simulink model "mech_stewart_trajectory"  (R2017a)
settings: Solver=ode45  StartTime=0.0  StopTime=inf  RelTol=1e-3  EnableMultiTasking=on
PreLoadFcn:
  | mech_stewartplatform_dat
PostLoadFcn:
  | find_system(gcs,'FollowLinks', 'on', 'LookUnderMasks', 'all');
InitFcn:
  | find_system(gcs,'FollowLinks', 'on', 'LookUnderMasks', 'all');
undefined symbols (not defined in the file): body_pts, height, Kd, Ki, Kp, lower_leg_mass, pos_base, pos_top, top_inertia, top_mass, upper_leg_mass
libraries: mblibv1 x9, mech_stewartplatform_leg x6
Description:
  | Stewart Platform with Control Reference Trajectory
  | 
  | This example shows a Stewart platform with predefined reference trajectory. A Stewart platform is a six-degree-of-freedom machine for precise positioning and orienting. It consists of a top plate connected to a fixed base through six parallel legs. By extending or shortening the legs and swiveling them on a set of universal joints, the plate's original six degrees of freedom are reproduced with greater stability and precision.
  | 
  | The model is separated into a plant subsystem, the Stewart platform along with necessary actuators and sensors, and a controller subsystem that guides the platform through a predefined motion profile with actuation signals. The controller keeps the actual motion close to the reference motion via sensor-actuator feedback.
  | 
  | 
  | Copyright 2008-2017 The MathWorks, Inc.
settings Model: FPTRunName=Active  ExtModeAutoUpdateStatusClock=off  Creator=MathWorks  LastModifiedBy=smiller
settings DataIOCC: LimitDataPoints=on  SaveFormat=Array  SignalLoggingSaveFormat=ModelDataLogs  SignalLoggingName=logsOut  OutputTimes=[0:0.01:50]
settings OptimizationCC: BooleanDataType=off  ExpressionDepthLimit=2147483647  InitFltsAndDblsToZero=on  LifeSpan=inf
settings DebuggingCC: UnderspecifiedInitializationDetection=Classic  MergeDetectMultiDrivingBlocksExec=none  CheckExecutionContextPreStartOutputMsg=on  CheckExecutionContextRuntimeOutputMsg=on  SignalResolutionControl=TryResolveAllWithWarning  MultiTaskDSMMsg=warning  MultiTaskCondExecSysMsg=none  SigSpecEnsureSampleTimeMsg=none  FcnCallInpInsideContextMsg=warning  StateNameClashWarn=warning  StrictBusMsg=None  SFUnexpectedBacktrackingDiag=warning  SFNoUnconditionalDefaultTransitionDiag=warning  SFExecutionAtInitializationDiag=none
settings HardwareCC: ProdBitPerPointer=32  ProdBitPerSizeT=32  ProdBitPerPtrDiffT=32  ProdLargestAtomicFloat=None  ProdIntDivRoundTo=Undefined  ProdEndianess=Unspecified  ProdWordSize=32  ProdHWDeviceType=32-bit Generic  TargetBitPerPointer=64  TargetBitPerSizeT=64  TargetBitPerPtrDiffT=64  TargetLongLongMode=on  TargetIntDivRoundTo=Zero  TargetEndianess=LittleEndian  TargetWordSize=64  TargetHWDeviceType=MATLAB Host  ProdEqTarget=off
settings ModelReferenceCC: PropagateSignalLabelsOutOfModel=off
settings GRTTargetCC: TargetLangStandard=C89/C90 (ANSI)  GeneratePreprocessorConditionals=Disable all  CombineOutputUpdateFcns=off  GRTInterface=on
settings ConfigComp: CovMetricSettings=dw  CovHtmlReporting=on  CovSaveCumulativeToWorkspaceVar=on  CovSaveSingleToWorkspaceVar=on  CovExternalEMLEnable=off
settings ConfigurationSet: Description=SimMechanics 2G

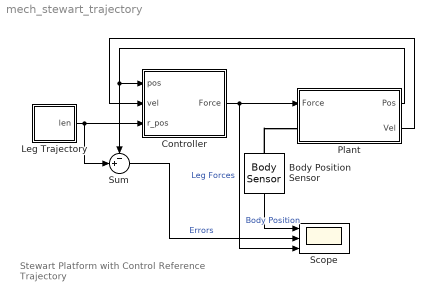
== system mech_stewart_trajectory ==
  note: Stewart Platform
      | with Control Reference Trajectory
  Body Position Sensor : mblibv1/Sensors &  Actuators/Body Sensor  UpdateFromCAD=off  PhysicalDomain=Mechanical  PortType=blob  Muxed=on  Pose=off  Angle=on  AngleUnits=deg  ArcVelocity=off  ArcVelocityUnits=deg/s  ArcAcceleration=off  ArcAccelerationUnits=deg/s^2  CoordPosition=on  CoordPositionUnits=m  Velocity=off  VelocityUnits=m/s  Acceleration=off  AccelerationUnits=m/s^2  Quaternion=on  QuaternionDT=off  QuaternionDDT=off  QuaternionUnits=off  OutputVector=[ 3 ]  ActiveIO=on  Width=3  DialogClass=MechanicalSensorBlock  ReferenceFrame=Absolute (World)
      settings: SourceProductName=Simscape Multibody  SourceProductBaseCode=MS
  Controller : Subsystem
  Leg Trajectory : Subsystem
  Plant : Subsystem
  Scope : Scope  NumInputPorts=3
      settings: Tag=OpenMeAtStartUp
  Sum : Sum  Inputs=-+|  SaturateOnIntegerOverflow=on  InputSameDT=on  OutDataTypeStr=Inherit: Same as first input
  wires:
  Plant/1(Pos) -> Sum/1, Controller/1(pos)
  Controller/1(Force) -> Plant/1(Force), Scope/3  "Leg Forces"
  Body Position Sensor/1 -> Scope/1  "Body Position"
  Sum/1 -> Scope/2  "Errors"
  Leg Trajectory/1(len) -> Controller/3(r_pos), Sum/2
  Plant/2(Vel) -> Controller/2(vel)
  connections:
  Body Position Sensor/LConn1 -- Plant/LConn1

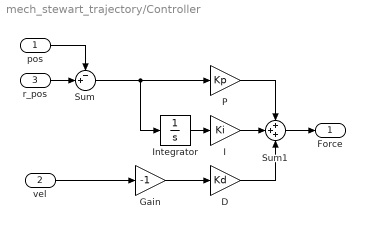
== system mech_stewart_trajectory/Controller ==
  pos : Inport
  vel : Inport  Port=2
  r_pos : Inport  Port=3
  D : Gain  Gain=Kd  SaturateOnIntegerOverflow=on  OutDataTypeStr=Inherit: Same as input  ParamDataTypeStr=Inherit: Same as input
  Gain : Gain  Gain=-1  SaturateOnIntegerOverflow=on  OutDataTypeStr=Inherit: Same as input  ParamDataTypeStr=Inherit: Same as input
  I : Gain  Gain=Ki  SaturateOnIntegerOverflow=on  OutDataTypeStr=Inherit: Same as input  ParamDataTypeStr=Inherit: Same as input
  Integrator : Integrator  InitialCondition=(upper_leg_mass+lower_leg_mass+(top_mass*1.3/6))*9.81/Ki  ZeroCross=off
  P : Gain  Gain=Kp  SaturateOnIntegerOverflow=on  OutDataTypeStr=Inherit: Same as input  ParamDataTypeStr=Inherit: Same as input
  Sum : Sum  Inputs=-+|  SaturateOnIntegerOverflow=on  InputSameDT=on  OutDataTypeStr=Inherit: Same as first input
  Sum1 : Sum  Inputs=+++  SaturateOnIntegerOverflow=on  InputSameDT=on  OutDataTypeStr=Inherit: Same as first input
  Force : Outport
  wires:
  Sum/1 -> P/1, Integrator/1
  I/1 -> Sum1/2
  P/1 -> Sum1/1
  Integrator/1 -> I/1
  vel/1 -> Gain/1
  D/1 -> Sum1/3
  pos/1 -> Sum/1
  Sum1/1 -> Force/1
  r_pos/1 -> Sum/2
  Gain/1 -> D/1

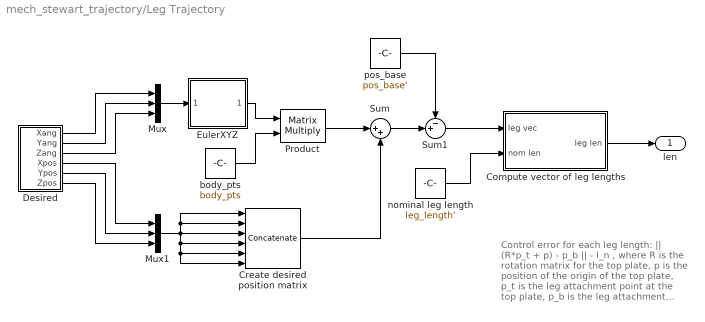
== system mech_stewart_trajectory/Leg Trajectory ==
  note: Control error for each leg length:
      |
      |   || (R*p_t + p) - p_b || - l_n ,
      |
      | where R is the rotation matrix
      | for the top plate, p is the position
      | of the origin of the top plate, p_t
      | is the leg attachment point at the
      | top plate, p_b is the leg attachment
      | point at the base, and l_n is the
      | nominal (reference) distance between
      | the top and base attachment points.
  Compute vector of leg lengths : Subsystem  TreatAsAtomicUnit=on
  Create desired position matrix : Concatenate  NumInputs=6  Mode=Multidimensional array  ConcatenateDimension=2
  Desired : Subsystem
  EulerXYZ : Subsystem  mask(EulerXYZ){}
      mask help: Creates the EulerXYZ rotation matrix corresponding to body fixed rotations in the X, Y, and then Z. This matrix maps body vectors to world vectors.
      mask Help:
      | <p>This block determines the EulerXYZ matrix from a 3x1 euler angles in the X, Y, & Z directions. The matrix maps vectors the body axes to the inertial axes.</p>
      | 
      | <p>The block input and output contain more than one signal as described below.</p>
      | 
      | <p><H4>Block Vector Input - Euler XYZ angles</H4>
      |     <ul>
      |     <li>X angle</li>
      |     <li>Y angle</li>
      |     <li>Z angle</li>
      |    </ul>
      |    </p>
      | 
      | <p><H4>Block Matrix Output - XYZ Euler Matrix </H4>
      |     <ul>
      |    </ul>
      |    </p>
      mask Display: disp('Rotation\nMatrix')
  Mux : Mux  Inputs=3
  Mux1 : Mux  Inputs=3
  Product : Product  Multiplication=Matrix(*)  SaturateOnIntegerOverflow=on  InputSameDT=on  OutDataTypeStr=Inherit: Same as first input
  Sum : Sum  Inputs=|++  SaturateOnIntegerOverflow=on  InputSameDT=on  OutDataTypeStr=Inherit: Same as first input
  Sum1 : Sum  Inputs=-+|  SaturateOnIntegerOverflow=on  InputSameDT=on  OutDataTypeStr=Inherit: Same as first input
  body_pts : Constant  Value=body_pts  VectorParams1D=off
  nominal leg length : Constant  Value=leg_length'  VectorParams1D=off
  pos_base : Constant  Value=pos_base'  VectorParams1D=off
  len : Outport
  wires:
  Mux/1 -> EulerXYZ/1(x y z angles)
  EulerXYZ/1(EulerXYZ) -> Product/1
  body_pts/1 -> Product/2
  Product/1 -> Sum/1
  Mux1/1 -> Create desired position matrix/3, Create desired position matrix/1, Create desired position matrix/2, Create desired position matrix/4, Create desired position matrix/5, Create desired position matrix/6
  Create desired position matrix/1 -> Sum/2
  pos_base/1 -> Sum1/1
  Sum/1 -> Sum1/2
  Sum1/1 -> Compute vector of leg lengths/1(leg vec)
  nominal leg length/1 -> Compute vector of leg lengths/2(nom len)
  Compute vector of leg lengths/1(leg len) -> len/1
  Desired/3(Zang) -> Mux/3
  Desired/1(Xang) -> Mux/1
  Desired/2(Yang) -> Mux/2
  Desired/4(Xpos) -> Mux1/1
  Desired/5(Ypos) -> Mux1/2
  Desired/6(Zpos) -> Mux1/3

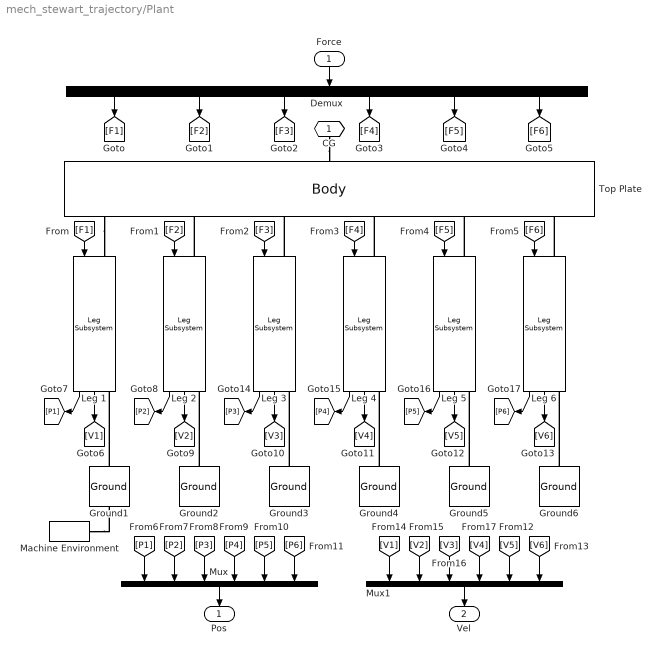
== system mech_stewart_trajectory/Plant ==
  Force : Inport
  Demux : Demux  Outputs=6
  Ground1 : mblibv1/Bodies/Ground  UpdateFromCAD=off  LeftPortType=env  RightPortType=workingframe  PhysicalDomain=Mechanical  DialogClass=GroundBlock  CoordPosition=pos_base(1,:)  CoordPositionUnits=m  StateVectorMgrId=-1  MachineId=[0 0]  ShowEnvPort=on  ParameterChecksum=[0 0 0 0]  TopologyChecksum=[0 0 0 0]
      settings: SourceProductName=Simscape Multibody  SourceProductBaseCode=MS
  Ground2 : mblibv1/Bodies/Ground  UpdateFromCAD=off  LeftPortType=env  RightPortType=workingframe  PhysicalDomain=Mechanical  DialogClass=GroundBlock  CoordPosition=pos_base(2,:)  CoordPositionUnits=m  StateVectorMgrId=-1  MachineId=[0 0]  ShowEnvPort=off  ParameterChecksum=[0 0 0 0]  TopologyChecksum=[0 0 0 0]
      settings: SourceProductName=Simscape Multibody  SourceProductBaseCode=MS
  Ground3 : mblibv1/Bodies/Ground  UpdateFromCAD=off  LeftPortType=env  RightPortType=workingframe  PhysicalDomain=Mechanical  DialogClass=GroundBlock  CoordPosition=pos_base(3,:)  CoordPositionUnits=m  StateVectorMgrId=-1  MachineId=[0 0]  ShowEnvPort=off  ParameterChecksum=[0 0 0 0]  TopologyChecksum=[0 0 0 0]
      settings: SourceProductName=Simscape Multibody  SourceProductBaseCode=MS
  Ground4 : mblibv1/Bodies/Ground  UpdateFromCAD=off  LeftPortType=env  RightPortType=workingframe  PhysicalDomain=Mechanical  DialogClass=GroundBlock  CoordPosition=pos_base(4,:)  CoordPositionUnits=m  StateVectorMgrId=-1  MachineId=[0 0]  ShowEnvPort=off  ParameterChecksum=[0 0 0 0]  TopologyChecksum=[0 0 0 0]
      settings: SourceProductName=Simscape Multibody  SourceProductBaseCode=MS
  Ground5 : mblibv1/Bodies/Ground  UpdateFromCAD=off  LeftPortType=env  RightPortType=workingframe  PhysicalDomain=Mechanical  DialogClass=GroundBlock  CoordPosition=pos_base(5,:)  CoordPositionUnits=m  StateVectorMgrId=-1  MachineId=[0 0]  ShowEnvPort=off  ParameterChecksum=[0 0 0 0]  TopologyChecksum=[0 0 0 0]
      settings: SourceProductName=Simscape Multibody  SourceProductBaseCode=MS
  Ground6 : mblibv1/Bodies/Ground  UpdateFromCAD=off  LeftPortType=env  RightPortType=workingframe  PhysicalDomain=Mechanical  DialogClass=GroundBlock  CoordPosition=pos_base(6,:)  CoordPositionUnits=m  StateVectorMgrId=-1  MachineId=[0 0]  ShowEnvPort=off  ParameterChecksum=[0 0 0 0]  TopologyChecksum=[0 0 0 0]
      settings: SourceProductName=Simscape Multibody  SourceProductBaseCode=MS
  Leg 1 : mech_stewartplatform_leg/Leg Subsystem  ln=1
  Leg 2 : mech_stewartplatform_leg/Leg Subsystem  ln=2
  Leg 3 : mech_stewartplatform_leg/Leg Subsystem  ln=3
  Leg 4 : mech_stewartplatform_leg/Leg Subsystem  ln=4
  Leg 5 : mech_stewartplatform_leg/Leg Subsystem  ln=5
  Leg 6 : mech_stewartplatform_leg/Leg Subsystem  ln=6
  Machine Environment : mblibv1/Bodies/Machine Environment  Tag=Factory ground  PortType=env  PhysicalDomain=Mechanical  DialogTemplateClass=MECH.MachineEnvironment  SyncWhenCopied=off  Gravity=[0 0 -9.81]  GravityUnits=m/s^2  GravityAsSignal=off  Dimensionality=3D Only  AnalysisType=Forward dynamics  LinearAssemblyTolerance=1e-3  LinearAssemblyToleranceUnits=m  AngularAssemblyTolerance=1e-3  AngularAssemblyToleranceUnits=rad  ConstraintSolverType=Machine precision  ConstraintRelTolerance=1e-4  ConstraintAbsTolerance=1e-4  UseRobustSingularityHandling=on  RedundancyAnalysisToleranceType=Automatically select tolerance  RedundancyAnalysisTolerance=1e-14  StatePerturbationType=Adaptive  PerturbationSize=1e-3  VisualizeMachine=on  BodyVisualizationType=Use model default body geometries  BodyColorSelMode=Use model default  DefaultBodyColor=[1 0 0]
      settings: SourceProductName=Simscape Multibody  SourceProductBaseCode=MS
  Mux : Mux  Inputs=6
  Mux1 : Mux  Inputs=6
  Top Plate : mblibv1/Bodies/Body  LConnTagsString=CG  RConnTagsString=CS1|CS2|CS3|CS4|CS5|CS6  UpdateFromCAD=off  DialogClass=MechanicalBodyBlock  Mass=top_mass  MassUnits=kg  InertiaUnits=kg*m^2  Inertia=top_inertia  Shape=Cylinder  ShapeDims=[1 1]  ShapeUnits=m  ShapeUse=false  Density=1  DensityUnits=kg/m^3  DensityUse=false  GraphicsMode=MACHINE_DEFAULT  BodyColorSelMode=MACHINE_DEFAULT  BodyColor=[1 0 0]  AttachedToCS=CG  CG=Left$CG$[0 0 height]$WORLD$WORLD$m$[0 0 0]$Euler X-Y-Z$deg$WORLD$true  WorkingFrames=Right$CS1$pos_top(1,:)$WORLD$WORLD$m$[0 0 0]$Euler X-Y-Z$deg$WORLD$true#Right$CS2$pos_top(2,:)$WORLD$WORLD$m$[0 0 0]$Euler X-Y-Z$deg$WORLD$true#Right$CS3$pos_top(3,:)$WORLD$WORLD$m$[0 0 0]$Euler X-Y-Z$deg$WORLD$true#Right$CS4$pos_top(4,:)$WORLD$WORLD$m$[0 0 0]$Euler X-Y-Z$deg$WORLD$true#Right$CS5$pos_top(5,:)$WORLD$WORLD$m$[0 0 0]$Euler X-Y-Z$deg$WORLD$true#Right$CS6$pos_top(6,:)$WORLD$WORLD$m$[0 0 0]$Euler X-Y-Z$deg$WORLD$true  CGPos=[0 0 height]  CGRot=[0 0 0]  CS0Pos=[]  CS0Rot=[]  CS1Pos=pos_top(1,:)  CS1Rot=[0 0 0]  CS2Pos=pos_top(2,:)  CS2Rot=[0 0 0]  CS3Pos=pos_top(3,:)  CS3Rot=[0 0 0]  CS4Pos=pos_top(4,:)  CS4Rot=[0 0 0]  CS5Pos=pos_top(5,:)  CS5Rot=[0 0 0]  CS6Pos=pos_top(6,:)  CS6Rot=[0 0 0]  CS7Pos=[]  CS7Rot=[]  CS8Pos=[]  CS8Rot=[]  CS9Pos=[]  CS9Rot=[]  CS10Pos=[]  CS10Rot=[]  CS11Pos=[]  CS11Rot=[]  CS12Pos=[]  CS12Rot=[]  CS13Pos=[]  CS13Rot=[]  CS14Pos=[]  CS14Rot=[]  CS15Pos=[]  CS15Rot=[]  CS16Pos=[]  CS16Rot=[]  CS17Pos=[]  CS17Rot=[]  CS18Pos=[]  CS18Rot=[]  CS19Pos=[]  CS19Rot=[]  CS20Pos=[]  CS20Rot=[]
      settings: SourceProductName=Simscape Multibody  SourceProductBaseCode=MS
  CG : PMIOPort  Port=1  Side=Left
  Pos : Outport
  Vel : Outport  Port=2
  wires:
  Force/1 -> Demux/1
  Mux/1 -> Pos/1
  Demux/1 -> [F1]
  Demux/2 -> [F2]
  Demux/3 -> [F3]
  Demux/4 -> [F4]
  Demux/5 -> [F5]
  Demux/6 -> [F6]
  [F1] -> Leg 1/1
  [F2] -> Leg 2/1
  [F3] -> Leg 3/1
  [F4] -> Leg 4/1
  [F5] -> Leg 5/1
  [F6] -> Leg 6/1
  Leg 1/2 -> [V1]
  Leg 1/1 -> [P1]
  Leg 2/2 -> [V2]
  Leg 3/2 -> [V3]
  Leg 4/2 -> [V4]
  Leg 5/2 -> [V5]
  Leg 6/2 -> [V6]
  Leg 2/1 -> [P2]
  Leg 3/1 -> [P3]
  Leg 4/1 -> [P4]
  Leg 5/1 -> [P5]
  Leg 6/1 -> [P6]
  [P1] -> Mux/1
  [P2] -> Mux/2
  [P3] -> Mux/3
  [P4] -> Mux/4
  [P5] -> Mux/5
  [P6] -> Mux/6
  [V1] -> Mux1/1
  [V2] -> Mux1/2
  [V3] -> Mux1/3
  [V4] -> Mux1/4
  [V5] -> Mux1/5
  [V6] -> Mux1/6
  Mux1/1 -> Vel/1
  connections:
  Top Plate/RConn1 -- Leg 1/LConn1
  Ground6/RConn1 -- Leg 6/RConn1
  Ground5/RConn1 -- Leg 5/RConn1
  Ground4/RConn1 -- Leg 4/RConn1
  Ground3/RConn1 -- Leg 3/RConn1
  Ground2/RConn1 -- Leg 2/RConn1
  Ground1/RConn1 -- Leg 1/RConn1
  Leg 2/LConn1 -- Top Plate/RConn2
  Leg 3/LConn1 -- Top Plate/RConn3
  Leg 4/LConn1 -- Top Plate/RConn4
  Leg 5/LConn1 -- Top Plate/RConn5
  Leg 6/LConn1 -- Top Plate/RConn6
  CG/RConn1 -- Top Plate/LConn1
  Machine Environment/RConn1 -- Ground1/LConn1

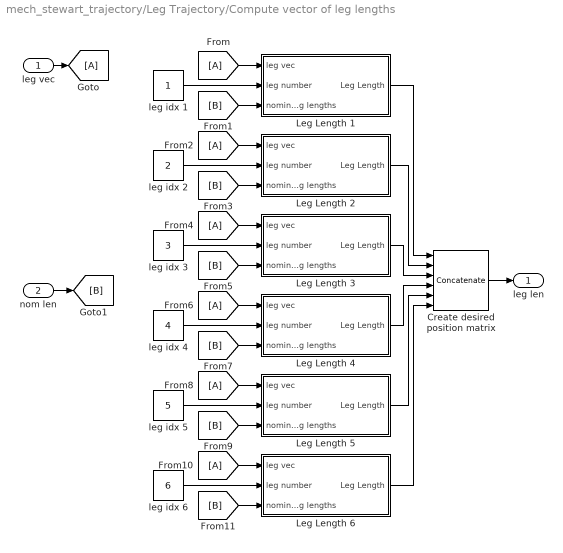
== system mech_stewart_trajectory/Leg Trajectory/Compute vector of leg lengths ==
  leg vec : Inport
  nom len : Inport  Port=2
  Create desired position matrix : Concatenate  NumInputs=6  Mode=Multidimensional array  ConcatenateDimension=2
  Leg Length 1 : Subsystem
  Leg Length 2 : Subsystem
  Leg Length 3 : Subsystem
  Leg Length 4 : Subsystem
  Leg Length 5 : Subsystem
  Leg Length 6 : Subsystem
  leg idx 1 : Constant
  leg idx 2 : Constant  Value=2
  leg idx 3 : Constant  Value=3
  leg idx 4 : Constant  Value=4
  leg idx 5 : Constant  Value=5
  leg idx 6 : Constant  Value=6
  leg len : Outport
  wires:
  Leg Length 6/1(Leg Length) -> Create desired position matrix/6
  Leg Length 5/1(Leg Length) -> Create desired position matrix/5
  Leg Length 4/1(Leg Length) -> Create desired position matrix/4
  Leg Length 3/1(Leg Length) -> Create desired position matrix/3
  Leg Length 2/1(Leg Length) -> Create desired position matrix/2
  Leg Length 1/1(Leg Length) -> Create desired position matrix/1
  [B] -> Leg Length 6/3(nominal leg lengths)
  [A] -> Leg Length 6/1(leg vec)
  leg idx 6/1 -> Leg Length 6/2(leg number)
  [B] -> Leg Length 5/3(nominal leg lengths)
  [A] -> Leg Length 5/1(leg vec)
  leg idx 5/1 -> Leg Length 5/2(leg number)
  [B] -> Leg Length 4/3(nominal leg lengths)
  [A] -> Leg Length 4/1(leg vec)
  leg idx 4/1 -> Leg Length 4/2(leg number)
  [B] -> Leg Length 3/3(nominal leg lengths)
  [A] -> Leg Length 3/1(leg vec)
  leg idx 3/1 -> Leg Length 3/2(leg number)
  [B] -> Leg Length 2/3(nominal leg lengths)
  [A] -> Leg Length 2/1(leg vec)
  leg idx 2/1 -> Leg Length 2/2(leg number)
  [B] -> Leg Length 1/3(nominal leg lengths)
  nom len/1 -> [B]
  [A] -> Leg Length 1/1(leg vec)
  leg vec/1 -> [A]
  leg idx 1/1 -> Leg Length 1/2(leg number)
  Create desired position matrix/1 -> leg len/1

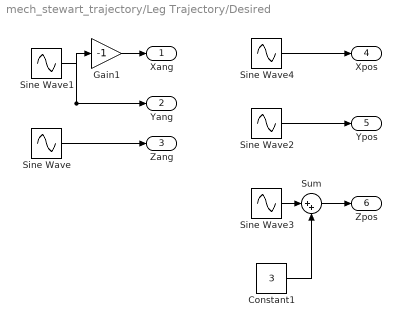
== system mech_stewart_trajectory/Leg Trajectory/Desired ==
  Constant1 : Constant  Value=3
  Gain1 : Gain  Gain=-1  SaturateOnIntegerOverflow=on  OutDataTypeStr=Inherit: Same as input  ParamDataTypeStr=Inherit: Same as input
  Sine Wave : Sin  Amplitude=0.3  Frequency=3  SampleTime=0
  Sine Wave1 : Sin  Amplitude=0.3  Frequency=3  SampleTime=0
  Sine Wave2 : Sin  Amplitude=0.25  Frequency=3  Phase=pi/2  SampleTime=0
  Sine Wave3 : Sin  Amplitude=0.25  Frequency=3  SampleTime=0
  Sine Wave4 : Sin  Amplitude=0.5  Frequency=3  SampleTime=0
  Sum : Sum  Inputs=|++  SaturateOnIntegerOverflow=on  InputSameDT=on  OutDataTypeStr=Inherit: Same as first input
  Xang : Outport
  Yang : Outport  Port=2
  Zang : Outport  Port=3
  Xpos : Outport  Port=4
  Ypos : Outport  Port=5
  Zpos : Outport  Port=6
  wires:
  Sine Wave/1 -> Zang/1
  Sine Wave1/1 -> Gain1/1, Yang/1
  Gain1/1 -> Xang/1
  Sine Wave2/1 -> Ypos/1
  Sine Wave3/1 -> Sum/1
  Sum/1 -> Zpos/1
  Constant1/1 -> Sum/2
  Sine Wave4/1 -> Xpos/1

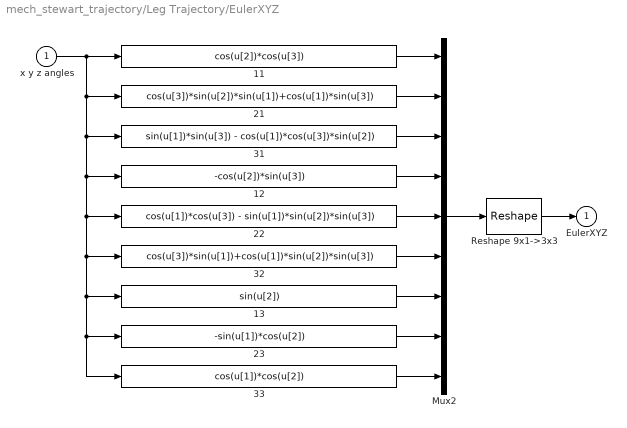
== system mech_stewart_trajectory/Leg Trajectory/EulerXYZ ==
  x y z angles : Inport
  11 : Fcn  Expr=cos(u[2])*cos(u[3])
  12 : Fcn  Expr=-cos(u[2])*sin(u[3])
  13 : Fcn  Expr=sin(u[2])
  21 : Fcn  Expr=cos(u[3])*sin(u[2])*sin(u[1])+cos(u[1])*sin(u[3])
  22 : Fcn  Expr=cos(u[1])*cos(u[3]) - sin(u[1])*sin(u[2])*sin(u[3])
  23 : Fcn  Expr=-sin(u[1])*cos(u[2])
  31 : Fcn  Expr=sin(u[1])*sin(u[3]) - cos(u[1])*cos(u[3])*sin(u[2])
  32 : Fcn  Expr=cos(u[3])*sin(u[1])+cos(u[1])*sin(u[2])*sin(u[3])
  33 : Fcn  Expr=cos(u[1])*cos(u[2])
  Mux2 : Mux  Inputs=9
  Reshape 9x1->3x3 : Reshape  OutputDimensionality=Customize  OutputDimensions=[3,3]
  EulerXYZ : Outport  InitialOutput=0
  wires:
  x y z angles/1 -> 23/1, 33/1, 13/1, 32/1, 22/1, 12/1, 31/1, 21/1, 11/1
  33/1 -> Mux2/9
  23/1 -> Mux2/8
  13/1 -> Mux2/7
  32/1 -> Mux2/6
  22/1 -> Mux2/5
  12/1 -> Mux2/4
  31/1 -> Mux2/3
  21/1 -> Mux2/2
  11/1 -> Mux2/1
  Mux2/1 -> Reshape 9x1->3x3/1
  Reshape 9x1->3x3/1 -> EulerXYZ/1

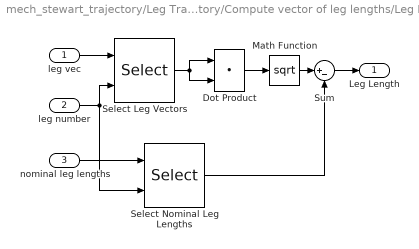
== system mech_stewart_trajectory/Leg Trajectory/Compute vector of leg lengths/Leg Length 1 ==
  leg vec : Inport
  leg number : Inport  Port=2
  nominal leg lengths : Inport  Port=3
  Dot Product : DotProduct  OutDataTypeStr=Inherit: Inherit via internal rule
  Math Function : Math  Operator=sqrt  SaturateOnIntegerOverflow=on
  Select Leg Vectors : Selector  NumberOfDimensions=2  InputPortWidth=3  IndexOptions=Select all,Index vector (port)  Indices=-1,1  OutputSizes=1
  Select Nominal Leg Lengths : Selector  InputPortWidth=6  IndexOptions=Index vector (port)  Indices=[1 3]  OutputSizes=1
  Sum : Sum  Inputs=|+-  SaturateOnIntegerOverflow=on  InputSameDT=on  OutDataTypeStr=Inherit: Same as first input
  Leg Length : Outport
  wires:
  nominal leg lengths/1 -> Select Nominal Leg Lengths/1
  Sum/1 -> Leg Length/1
  leg vec/1 -> Select Leg Vectors/1
  leg number/1 -> Select Leg Vectors/2, Select Nominal Leg Lengths/2
  Dot Product/1 -> Math Function/1
  Select Leg Vectors/1 -> Dot Product/1, Dot Product/2
  Math Function/1 -> Sum/1
  Select Nominal Leg Lengths/1 -> Sum/2

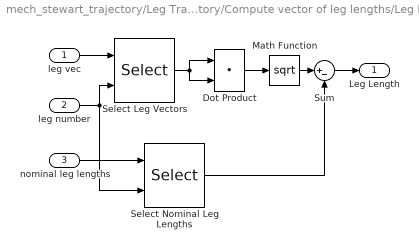
== system mech_stewart_trajectory/Leg Trajectory/Compute vector of leg lengths/Leg Length 2 ==
  leg vec : Inport
  leg number : Inport  Port=2
  nominal leg lengths : Inport  Port=3
  Dot Product : DotProduct  OutDataTypeStr=Inherit: Inherit via internal rule
  Math Function : Math  Operator=sqrt  SaturateOnIntegerOverflow=on
  Select Leg Vectors : Selector  NumberOfDimensions=2  InputPortWidth=3  IndexOptions=Select all,Index vector (port)  Indices=-1,1  OutputSizes=1
  Select Nominal Leg Lengths : Selector  InputPortWidth=6  IndexOptions=Index vector (port)  Indices=[1 3]  OutputSizes=1
  Sum : Sum  Inputs=|+-  SaturateOnIntegerOverflow=on  InputSameDT=on  OutDataTypeStr=Inherit: Same as first input
  Leg Length : Outport
  wires:
  nominal leg lengths/1 -> Select Nominal Leg Lengths/1
  Sum/1 -> Leg Length/1
  leg vec/1 -> Select Leg Vectors/1
  leg number/1 -> Select Leg Vectors/2, Select Nominal Leg Lengths/2
  Dot Product/1 -> Math Function/1
  Select Leg Vectors/1 -> Dot Product/1, Dot Product/2
  Math Function/1 -> Sum/1
  Select Nominal Leg Lengths/1 -> Sum/2

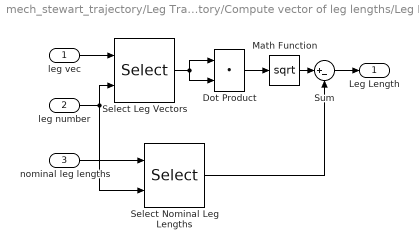
== system mech_stewart_trajectory/Leg Trajectory/Compute vector of leg lengths/Leg Length 3 ==
  leg vec : Inport
  leg number : Inport  Port=2
  nominal leg lengths : Inport  Port=3
  Dot Product : DotProduct  OutDataTypeStr=Inherit: Inherit via internal rule
  Math Function : Math  Operator=sqrt  SaturateOnIntegerOverflow=on
  Select Leg Vectors : Selector  NumberOfDimensions=2  InputPortWidth=3  IndexOptions=Select all,Index vector (port)  Indices=-1,1  OutputSizes=1
  Select Nominal Leg Lengths : Selector  InputPortWidth=6  IndexOptions=Index vector (port)  Indices=[1 3]  OutputSizes=1
  Sum : Sum  Inputs=|+-  SaturateOnIntegerOverflow=on  InputSameDT=on  OutDataTypeStr=Inherit: Same as first input
  Leg Length : Outport
  wires:
  nominal leg lengths/1 -> Select Nominal Leg Lengths/1
  Sum/1 -> Leg Length/1
  leg vec/1 -> Select Leg Vectors/1
  leg number/1 -> Select Leg Vectors/2, Select Nominal Leg Lengths/2
  Dot Product/1 -> Math Function/1
  Select Leg Vectors/1 -> Dot Product/1, Dot Product/2
  Math Function/1 -> Sum/1
  Select Nominal Leg Lengths/1 -> Sum/2

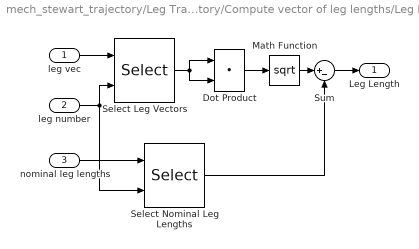
== system mech_stewart_trajectory/Leg Trajectory/Compute vector of leg lengths/Leg Length 4 ==
  leg vec : Inport
  leg number : Inport  Port=2
  nominal leg lengths : Inport  Port=3
  Dot Product : DotProduct  OutDataTypeStr=Inherit: Inherit via internal rule
  Math Function : Math  Operator=sqrt  SaturateOnIntegerOverflow=on
  Select Leg Vectors : Selector  NumberOfDimensions=2  InputPortWidth=3  IndexOptions=Select all,Index vector (port)  Indices=-1,1  OutputSizes=1
  Select Nominal Leg Lengths : Selector  InputPortWidth=6  IndexOptions=Index vector (port)  Indices=[1 3]  OutputSizes=1
  Sum : Sum  Inputs=|+-  SaturateOnIntegerOverflow=on  InputSameDT=on  OutDataTypeStr=Inherit: Same as first input
  Leg Length : Outport
  wires:
  nominal leg lengths/1 -> Select Nominal Leg Lengths/1
  Sum/1 -> Leg Length/1
  leg vec/1 -> Select Leg Vectors/1
  leg number/1 -> Select Leg Vectors/2, Select Nominal Leg Lengths/2
  Dot Product/1 -> Math Function/1
  Select Leg Vectors/1 -> Dot Product/1, Dot Product/2
  Math Function/1 -> Sum/1
  Select Nominal Leg Lengths/1 -> Sum/2

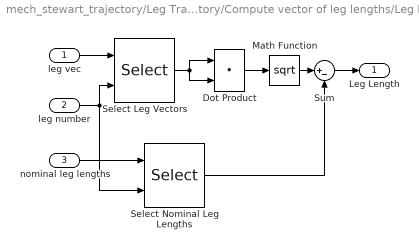
== system mech_stewart_trajectory/Leg Trajectory/Compute vector of leg lengths/Leg Length 5 ==
  leg vec : Inport
  leg number : Inport  Port=2
  nominal leg lengths : Inport  Port=3
  Dot Product : DotProduct  OutDataTypeStr=Inherit: Inherit via internal rule
  Math Function : Math  Operator=sqrt  SaturateOnIntegerOverflow=on
  Select Leg Vectors : Selector  NumberOfDimensions=2  InputPortWidth=3  IndexOptions=Select all,Index vector (port)  Indices=-1,1  OutputSizes=1
  Select Nominal Leg Lengths : Selector  InputPortWidth=6  IndexOptions=Index vector (port)  Indices=[1 3]  OutputSizes=1
  Sum : Sum  Inputs=|+-  SaturateOnIntegerOverflow=on  InputSameDT=on  OutDataTypeStr=Inherit: Same as first input
  Leg Length : Outport
  wires:
  nominal leg lengths/1 -> Select Nominal Leg Lengths/1
  Sum/1 -> Leg Length/1
  leg vec/1 -> Select Leg Vectors/1
  leg number/1 -> Select Leg Vectors/2, Select Nominal Leg Lengths/2
  Dot Product/1 -> Math Function/1
  Select Leg Vectors/1 -> Dot Product/1, Dot Product/2
  Math Function/1 -> Sum/1
  Select Nominal Leg Lengths/1 -> Sum/2

== system mech_stewart_trajectory/Leg Trajectory/Compute vector of leg lengths/Leg Length 6 ==
  leg vec : Inport
  leg number : Inport  Port=2
  nominal leg lengths : Inport  Port=3
  Dot Product : DotProduct  OutDataTypeStr=Inherit: Inherit via internal rule
  Math Function : Math  Operator=sqrt  SaturateOnIntegerOverflow=on
  Select Leg Vectors : Selector  NumberOfDimensions=2  InputPortWidth=3  IndexOptions=Select all,Index vector (port)  Indices=-1,1  OutputSizes=1
  Select Nominal Leg Lengths : Selector  InputPortWidth=6  IndexOptions=Index vector (port)  Indices=[1 3]  OutputSizes=1
  Sum : Sum  Inputs=|+-  SaturateOnIntegerOverflow=on  InputSameDT=on  OutDataTypeStr=Inherit: Same as first input
  Leg Length : Outport
  wires:
  nominal leg lengths/1 -> Select Nominal Leg Lengths/1
  Sum/1 -> Leg Length/1
  leg vec/1 -> Select Leg Vectors/1
  leg number/1 -> Select Leg Vectors/2, Select Nominal Leg Lengths/2
  Dot Product/1 -> Math Function/1
  Select Leg Vectors/1 -> Dot Product/1, Dot Product/2
  Math Function/1 -> Sum/1
  Select Nominal Leg Lengths/1 -> Sum/2
